simulink model "Qudcopter"  (R2021a)
settings: Solver=VariableStepAuto  StartTime=0.0  StopTime=40  RelTol=1e-3
values from neighbouring files (symbols this model uses):
  CS =     [CS.mat]    (also in Quad_dynamics.m = block.DialogPrm(1).Data)
libraries: simulink_extras x3, simulink x1
settings Model: Creator=gulso  LastModifiedBy=gulso
settings DataIOCC: SaveFormat=Structure  SignalLogging=off  DSMLogging=off  ReturnWorkspaceOutputs=off

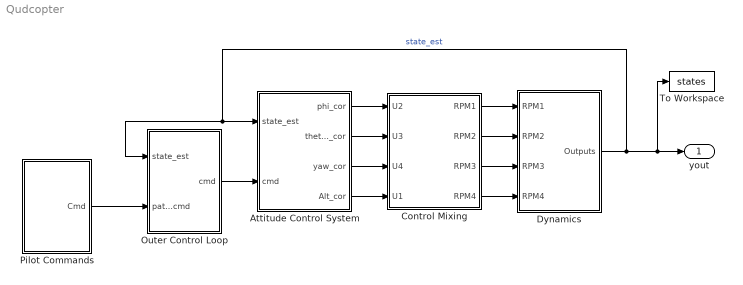
== system Qudcopter ==
  Attitude Control System : Subsystem
  "Control Mixing " : Subsystem
  Dynamics : Subsystem
  Outer Control Loop : Subsystem  mask{Kp=0.32, Ki=0.01, Kd=0.05}
      mask TypeOptions Kp: Kp1/Gain
      mask TypeOptions Ki: Ki/Gain
      mask TypeOptions Kd: Kd1/Gain
  Pilot Commands : Subsystem
  To Workspace : ToWorkspace  VariableName=states  SaveFormat=Timeseries  SampleTime=-1
      settings: Save2DSignal=2-D array (concatenate along first dimension)
  yout : Outport
  wires:
  Attitude Control System/3(yaw_cor) -> "Control Mixing "/3(U4)
  Attitude Control System/1(phi_cor) -> "Control Mixing "/1(U2)
  "Control Mixing "/3(RPM3) -> Dynamics/3(RPM3)
  Dynamics/1(Outputs) -> Attitude Control System/1(state_est), Outer Control Loop/1(state_est), yout/1, To Workspace/1  "state_est"
  "Control Mixing "/4(RPM4) -> Dynamics/4(RPM4)
  "Control Mixing "/2(RPM2) -> Dynamics/2(RPM2)
  "Control Mixing "/1(RPM1) -> Dynamics/1(RPM1)
  Outer Control Loop/1(cmd) -> Attitude Control System/2(cmd)
  Pilot Commands/1(Cmd) -> Outer Control Loop/2(path_cmd)
  Attitude Control System/2(theta_cor) -> "Control Mixing "/2(U3)
  Attitude Control System/4(Alt_cor) -> "Control Mixing "/4(U1)

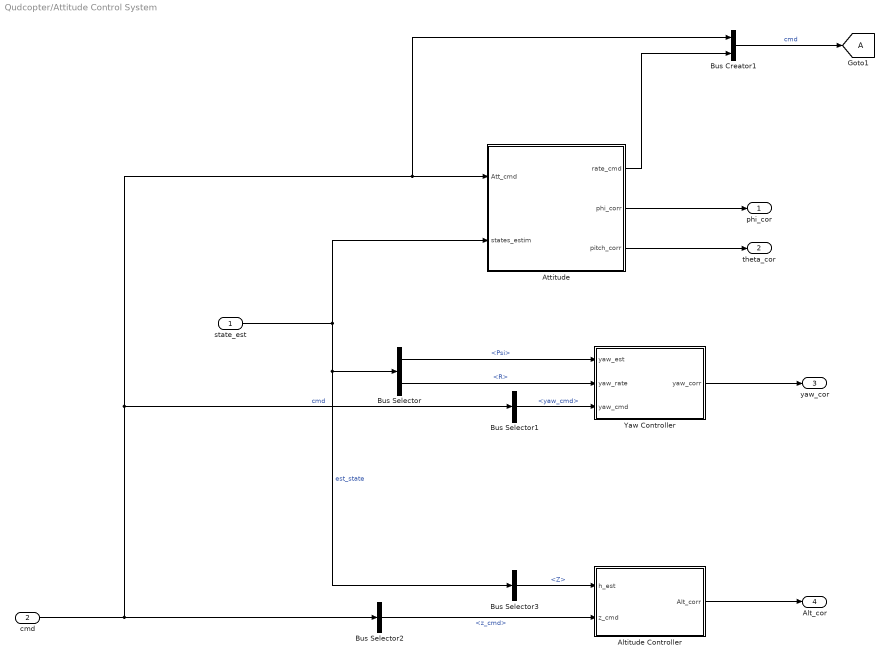
== system Qudcopter/Attitude Control System ==
  state_est : Inport
  cmd : Inport  Port=2
  Altitude Controller : Subsystem  mask{Kp=10, Ki=4, Kd=8}
      mask TypeOptions Kp: Gain/Gain
      mask TypeOptions Ki: Gain1/Gain
      mask TypeOptions Kd: Gain2/Gain
  Attitude : Subsystem  mask{Kp=2.4, Ki=1.1, Kd=1.8, Ki2=0.5}
      mask TypeOptions Kp: Kp1/Gain
      mask TypeOptions Ki: Ki1/Gain
      mask TypeOptions Kd: Kd1/Gain
      mask TypeOptions Ki2: Gainki/Gain
  Bus Creator1 : BusCreator  Inputs=2
  Bus Selector : BusSelector  OutputSignals=Psi,R
  Bus Selector1 : BusSelector  OutputSignals=pos_cmd.yaw_cmd
  Bus Selector2 : BusSelector  OutputSignals=pos_cmd.z_cmd
  Bus Selector3 : BusSelector  OutputSignals=Z
  Yaw Controller : Subsystem  mask{Kp=12, Ki=4, Kd=6}
      mask TypeOptions Kp: Gain/Gain
      mask TypeOptions Ki: Gain1/Gain
      mask TypeOptions Kd: Gain2/Gain
  phi_cor : Outport
  theta_cor : Outport  Port=2
  yaw_cor : Outport  Port=3
  Alt_cor : Outport  Port=4
  tag scope: A=global
  wires:
  Altitude Controller/1(Alt_corr) -> Alt_cor/1
  state_est/1 -> Attitude/2(states_estim), Bus Selector3/1, Bus Selector/1  "est_state"
  Bus Selector/1 -> Yaw Controller/1(yaw_est)  "<Psi>"
  Bus Selector/2 -> Yaw Controller/2(yaw_rate)  "<R>"
  cmd/1 -> Bus Selector2/1, Bus Creator1/1, Attitude/1(Att_cmd), Bus Selector1/1  "cmd"
  Bus Selector1/1 -> Yaw Controller/3(yaw_cmd)  "<yaw_cmd>"
  Bus Selector2/1 -> Altitude Controller/2(z_cmd)  "<z_cmd>"
  Bus Selector3/1 -> Altitude Controller/1(h_est)  "<Z>"
  Attitude/1(rate_cmd) -> Bus Creator1/2
  Attitude/2(phi_corr) -> phi_cor/1
  Attitude/3(pitch_corr) -> theta_cor/1
  Yaw Controller/1(yaw_corr) -> yaw_cor/1
  Bus Creator1/1 -> [A]  "cmd"

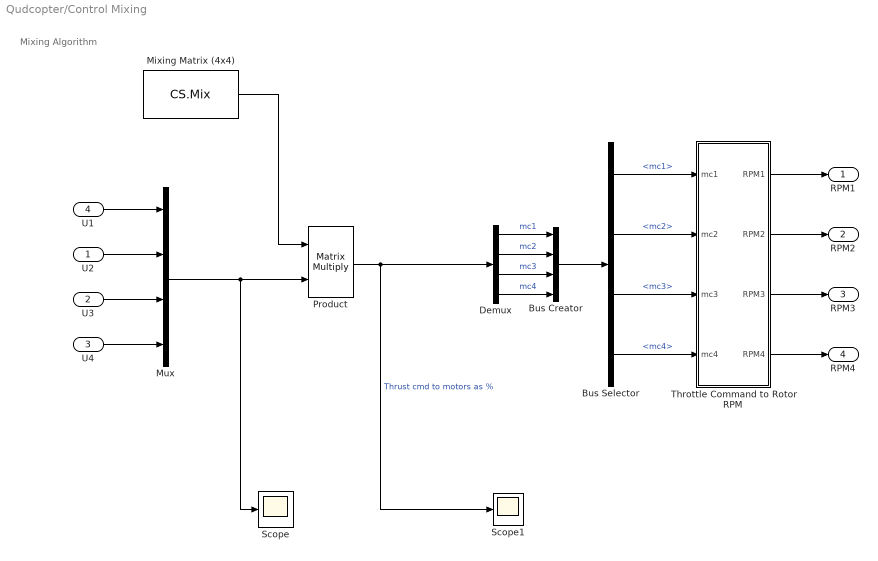
== system Qudcopter/Control Mixing  ==
  note: Mixing Algorithm
  U2 : Inport
  U3 : Inport  Port=2
  U4 : Inport  Port=3
  U1 : Inport  Port=4
  Bus Creator : BusCreator  Inputs=4
  Bus Selector : BusSelector  OutputSignals=mc1,mc2,mc3,mc4
  Demux : Demux
  Mixing Matrix (4x4) : Constant  Value=CS.Mix  OutDataTypeStr=single
  Mux : Mux
  Product : Product  Multiplication=Matrix(*)  RndMeth=Zero
  Scope : Scope
  Scope1 : Scope
  Throttle Command to Rotor RPM : Subsystem
  RPM1 : Outport
  RPM2 : Outport  Port=2
  RPM3 : Outport  Port=3
  RPM4 : Outport  Port=4
  wires:
  Throttle Command to Rotor RPM/4(RPM4) -> RPM4/1
  Throttle Command to Rotor RPM/3(RPM3) -> RPM3/1
  Throttle Command to Rotor RPM/1(RPM1) -> RPM1/1
  Throttle Command to Rotor RPM/2(RPM2) -> RPM2/1
  Bus Selector/4 -> Throttle Command to Rotor RPM/4(mc4)  "<mc4>"
  Product/1 -> Demux/1, Scope1/1  "Thrust cmd to motors as %"
  Demux/3 -> Bus Creator/3  "mc3"
  U2/1 -> Mux/2
  Mixing Matrix (4x4)/1 -> Product/1
  Bus Selector/1 -> Throttle Command to Rotor RPM/1(mc1)  "<mc1>"
  U3/1 -> Mux/3
  Demux/1 -> Bus Creator/1  "mc1"
  Demux/4 -> Bus Creator/4  "mc4"
  Bus Selector/3 -> Throttle Command to Rotor RPM/3(mc3)  "<mc3>"
  U4/1 -> Mux/4
  Demux/2 -> Bus Creator/2  "mc2"
  Bus Selector/2 -> Throttle Command to Rotor RPM/2(mc2)  "<mc2>"
  Bus Creator/1 -> Bus Selector/1
  U1/1 -> Mux/1
  Mux/1 -> Scope/1, Product/2

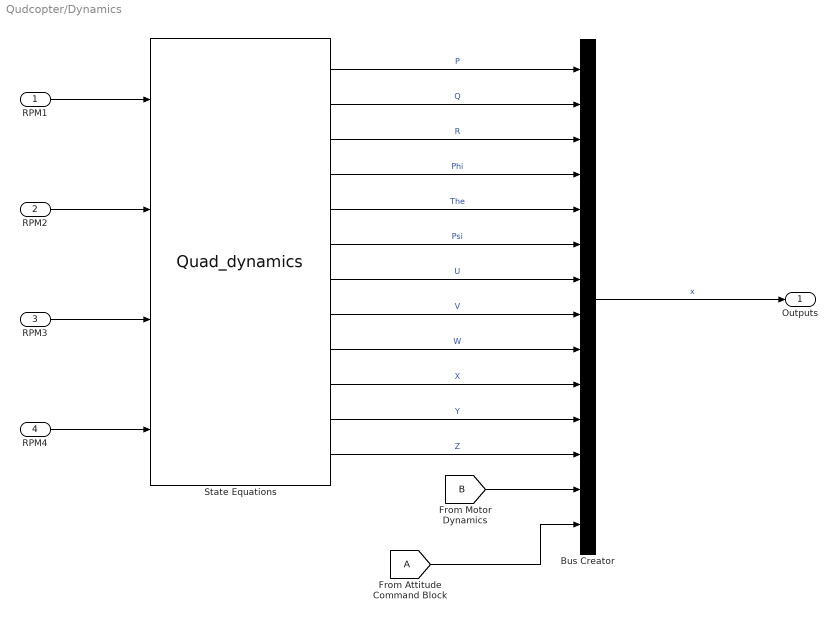
== system Qudcopter/Dynamics ==
  RPM1 : Inport
  RPM2 : Inport  Port=2
  RPM3 : Inport  Port=3
  RPM4 : Inport  Port=4
  Bus Creator : BusCreator  Inputs=14
  State Equations : M-S-Function  FunctionName=Quad_dynamics  Parameters=CS
      mask Display:
      | port_label('input', 1, 'RPM1')
      | port_label('input', 2, 'RPM2')
      | port_label('input', 3, 'RPM3')
      | port_label('input', 4, 'RPM4')
      | port_label('output', 1, 'P')
      | port_label('output', 2, 'Q')
      | port_label('output', 3, 'R')
      | port_label('output', 4, 'Phi')
      | port_label('output', 5, 'The')
      | port_label('output', 6, 'Psi')
      | port_label('output', 7, 'U')
      | port_label('output', 8, 'V')
      | port_label('output', 9, 'W')
      | port_label('output', 10, 'X')
      | port_label('output', 11, 'Y')
      | port_label('output', 12, 'Z')
  Outputs : Outport
  wires:
  State Equations/3 -> Bus Creator/3  "R"
  State Equations/1 -> Bus Creator/1  "P"
  State Equations/10 -> Bus Creator/10  "X"
  State Equations/5 -> Bus Creator/5  "The"
  State Equations/2 -> Bus Creator/2  "Q"
  State Equations/6 -> Bus Creator/6  "Psi"
  State Equations/7 -> Bus Creator/7  "U"
  State Equations/4 -> Bus Creator/4  "Phi"
  State Equations/11 -> Bus Creator/11  "Y"
  State Equations/9 -> Bus Creator/9  "W"
  State Equations/8 -> Bus Creator/8  "V"
  [B] -> Bus Creator/13
  Bus Creator/1 -> Outputs/1  "x"
  [A] -> Bus Creator/14
  State Equations/12 -> Bus Creator/12  "Z"
  RPM1/1 -> State Equations/1
  RPM2/1 -> State Equations/2
  RPM3/1 -> State Equations/3
  RPM4/1 -> State Equations/4

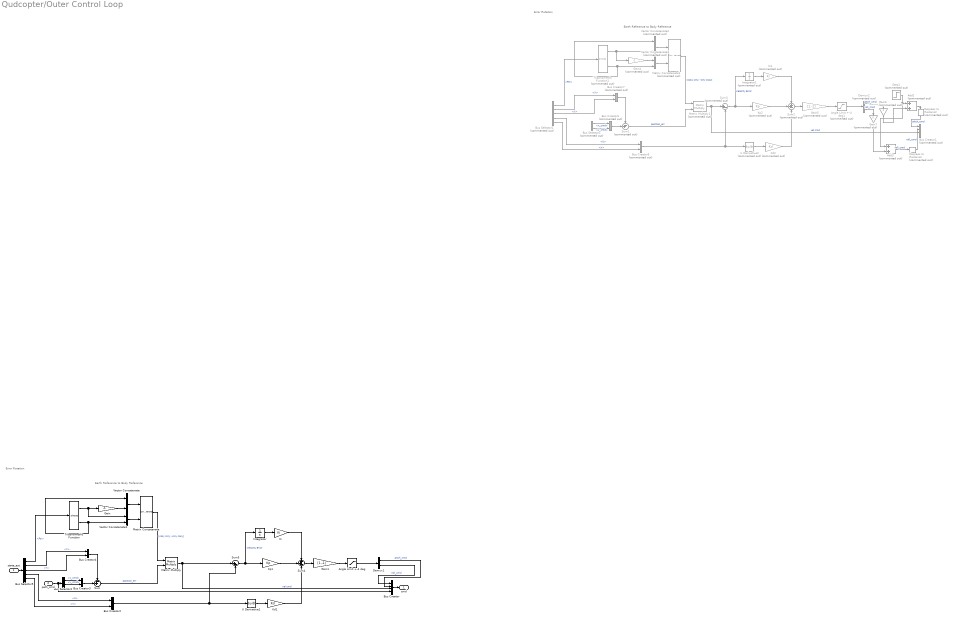
== system Qudcopter/Outer Control Loop ==
  note: Earth Reference to Body Reference
  note: Error Rotation
  note: Error Rotation
  note: Earth Reference to Body Reference
  state_est : Inport
  path_cmd : Inport  Port=2
  Add2 : Sum  Commented=on
  Add3 : Sum  Commented=on
  Angle Limit +-4 deg : Saturate  UpperLimit=4*pi/180  LowerLimit=-4*pi/180
  Angle Limit +-4 deg1 : Saturate  Commented=on  UpperLimit=4*pi/180  LowerLimit=-4*pi/180
  Bus Creator : BusCreator  Inputs=4
  Bus Creator1 : BusCreator  Commented=on  Inputs=4
  Bus Creator2 : BusCreator  Inputs=2
  Bus Creator3 : BusCreator  Inputs=2
  Bus Creator4 : BusCreator  Inputs=2
  Bus Creator5 : BusCreator  Commented=on  Inputs=2
  Bus Creator6 : BusCreator  Commented=on  Inputs=2
  Bus Creator7 : BusCreator  Commented=on  Inputs=2
  Bus Selector1 : BusSelector  Commented=on  OutputSignals=x_cmd,y_cmd
  Bus Selector2 : BusSelector  Commented=on  OutputSignals=Psi,X,Y,U,V
  Bus Selector4 : BusSelector  OutputSignals=x_cmd,y_cmd
  Bus Selector5 : BusSelector  OutputSignals=Psi,X,Y,U,V
  Degrees to Radians2 : simulink_extras/Transformations/Degrees to Radians  Commented=on
  Degrees to Radians3 : simulink_extras/Transformations/Degrees to Radians  Commented=on
  Demux1 : Demux  Outputs=2
  Demux2 : Demux  Commented=on  Outputs=2
  Gain : Gain  Gain=-1
  Gain1 : Gain  Gain=[1,-1]
  Gain4 : Gain  Commented=on  Gain=-1
  Gain5 : Gain  Commented=on  Gain=[1,-1]
  Gain6 : Gain  Commented=on  Gain=0
  Gain7 : Gain  Commented=on  Gain=0
  Integrator : Integrator  LimitOutput=on  UpperSaturationLimit=1  LowerSaturationLimit=-1
  Integrator1 : Integrator  Commented=on  LimitOutput=on  UpperSaturationLimit=1  LowerSaturationLimit=-1
  Kd1 : Gain  Gain=Kd
  Kd2 : Gain  Commented=on  Gain=Kd
  Ki : Gain  Gain=Ki
  Ki1 : Gain  Commented=on  Gain=Ki
  Kp1 : Gain  Gain=Kp
  Kp2 : Gain  Commented=on  Gain=Kp
  Matrix Concatenate : Concatenate  Mode=Multidimensional array  ConcatenateDimension=2
  Matrix Concatenate1 : Concatenate  Commented=on  Mode=Multidimensional array  ConcatenateDimension=2
  Matrix Multiply : Product  Multiplication=Matrix(*)
  Matrix Multiply1 : Product  Commented=on  Multiplication=Matrix(*)
  Step1 : Step  Commented=on  SampleTime=0
  Sum : Sum  Inputs=-+|
  Sum1 : Sum  Commented=on  Inputs=-+|
  Sum2 : Sum  Commented=on  Inputs=++-
  Sum3 : Sum  Commented=on  Inputs=|+-
  Sum4 : Sum  Inputs=++-
  Sum5 : Sum  Inputs=|+-
  Trigonometric Function : Trigonometry  Operator=sincos
  Trigonometric Function1 : Trigonometry  Commented=on  Operator=sincos
  U Derivative1 : Derivative
  U Derivative2 : Derivative  Commented=on
  Vector Concatenate : Concatenate
  Vector Concatenate1 : Concatenate
  Vector Concatenate2 : Concatenate  Commented=on
  Vector Concatenate3 : Concatenate  Commented=on
  cmd : Outport
  wires:
  Bus Selector5/1 -> Trigonometric Function/1  "<Psi>"
  state_est/1 -> Bus Selector5/1
  Bus Selector5/2 -> Bus Creator4/1  "<X>"
  Bus Selector5/5 -> Bus Creator2/2  "<V>"
  Bus Selector4/1 -> Bus Creator3/1  "<x_cmd>"
  Demux1/2 -> Bus Creator/1  "roll_cmd"
  Bus Selector4/2 -> Bus Creator3/2  "<y_cmd>"
  Bus Selector5/4 -> Bus Creator2/1  "<U>"
  Bus Selector5/3 -> Bus Creator4/2  "<Y>"
  path_cmd/1 -> Bus Creator/4, Bus Selector4/1
  Matrix Multiply/1 -> Bus Creator/3, Sum5/1  "vel cmd"
  Bus Creator/1 -> cmd/1
  Kp1/1 -> Sum4/2
  Sum5/1 -> Integrator/1, Kp1/1  "Velocity Error"
  Sum/1 -> Matrix Multiply/2  "position_err"
  Ki/1 -> Sum4/1
  Integrator/1 -> Ki/1
  Angle Limit +-4 deg/1 -> Demux1/1
  Gain1/1 -> Angle Limit +-4 deg/1
  Sum4/1 -> Gain1/1
  Kd1/1 -> Sum4/3
  Bus Creator2/1 -> U Derivative1/1, Sum5/2
  U Derivative1/1 -> Kd1/1
  Bus Creator4/1 -> Sum/1
  Bus Creator3/1 -> Sum/2
  Vector Concatenate/1 -> Matrix Concatenate/1
  Vector Concatenate1/1 -> Matrix Concatenate/2
  Trigonometric Function/1 -> Vector Concatenate1/1, Gain/1
  Matrix Concatenate/1 -> Matrix Multiply/1  "[cosy siny; -siny cosy]"
  Trigonometric Function/2 -> Vector Concatenate1/2, Vector Concatenate/1
  Gain6/1 -> Add2/2
  Add2/1 -> Degrees to Radians2/1
  Demux2/1 -> Gain6/1  "pitch_cmd"
  Add3/1 -> Degrees to Radians3/1  "roll_cmd"
  Demux2/2 -> Gain7/1  "roll_cmd"
  Trigonometric Function1/1 -> Vector Concatenate2/2, Gain4/1
  Trigonometric Function1/2 -> Vector Concatenate3/2, Vector Concatenate2/1
  Vector Concatenate2/1 -> Matrix Concatenate1/1
  Bus Creator6/1 -> Sum1/2
  Step1/1 -> Add3/1, Add2/1
  Bus Creator7/1 -> Sum1/1
  ? -> Bus Creator1/4, Bus Selector1/1
  Integrator1/1 -> Ki1/1
  Matrix Concatenate1/1 -> Matrix Multiply1/1  "[cosy siny; -siny cosy]"
  Kd2/1 -> Sum2/3
  Bus Creator5/1 -> U Derivative2/1, Sum3/2
  Bus Selector2/4 -> Bus Creator5/1  "<U>"
  Angle Limit +-4 deg1/1 -> Demux2/1
  Sum2/1 -> Gain5/1
  Degrees to Radians2/1 -> Bus Creator1/1  "pitch_cmd"
  Gain5/1 -> Angle Limit +-4 deg1/1
  Vector Concatenate3/1 -> Matrix Concatenate1/2
  Bus Selector2/3 -> Bus Creator7/2  "<Y>"
  Ki1/1 -> Sum2/1
  Sum1/1 -> Matrix Multiply1/2  "position_err"
  Sum3/1 -> Integrator1/1, Kp2/1  "Velocity Error"
  Gain7/1 -> Add3/2
  Matrix Multiply1/1 -> Bus Creator1/3, Sum3/1  "vel cmd"
  U Derivative2/1 -> Kd2/1
  Bus Selector2/1 -> Trigonometric Function1/1  "<Psi>"
  Kp2/1 -> Sum2/2
  Gain4/1 -> Vector Concatenate3/1
  Bus Selector2/5 -> Bus Creator5/2  "<V>"
  Bus Selector1/2 -> Bus Creator6/2  "<y_cmd>"
  Degrees to Radians3/1 -> Bus Creator1/2  "roll_cmd"
  ? -> Bus Selector2/1
  Bus Selector1/1 -> Bus Creator6/1  "<x_cmd>"
  Bus Selector2/2 -> Bus Creator7/1  "<X>"
  Demux1/1 -> Bus Creator/2  "pitch_cmd"
  Gain/1 -> Vector Concatenate/2

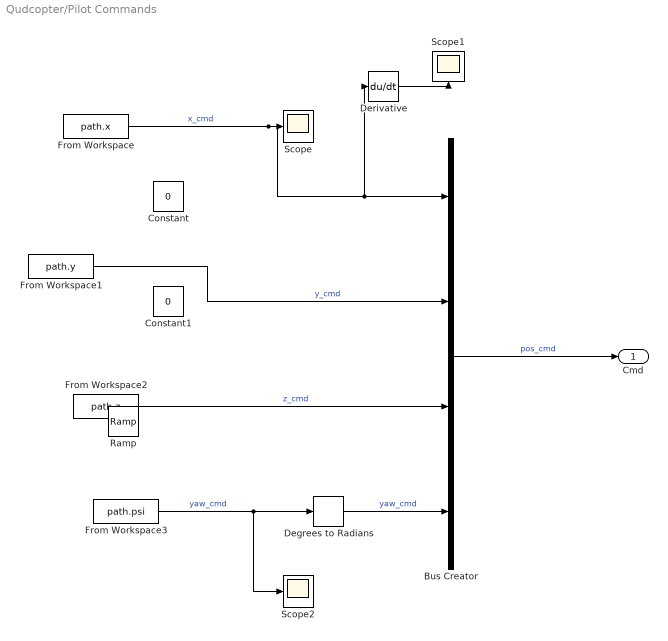
== system Qudcopter/Pilot Commands ==
  Bus Creator : BusCreator  Inputs=4
  Constant : Constant  Value=0
  Constant1 : Constant  Value=0
  Degrees to Radians : simulink_extras/Transformations/Degrees to Radians
  Derivative : Derivative
  From Workspace : FromWorkspace  VariableName=path.x
  From Workspace1 : FromWorkspace  VariableName=path.y
  From Workspace2 : FromWorkspace  VariableName=path.z
  From Workspace3 : FromWorkspace  VariableName=path.psi
  Ramp : simulink/Sources/Ramp  slope=1  start=0  InitialOutput=0
  Scope : Scope
  Scope1 : Scope
  Scope2 : Scope
  Cmd : Outport
  wires:
  Bus Creator/1 -> Cmd/1  "pos_cmd"
  Degrees to Radians/1 -> Bus Creator/4  "yaw_cmd"
  From Workspace/1 -> Derivative/1, Bus Creator/1, Scope/1  "x_cmd"
  From Workspace1/1 -> Bus Creator/2  "y_cmd"
  Derivative/1 -> Scope1/1
  From Workspace3/1 -> Scope2/1, Degrees to Radians/1  "yaw_cmd"
  From Workspace2/1 -> Bus Creator/3  "z_cmd"

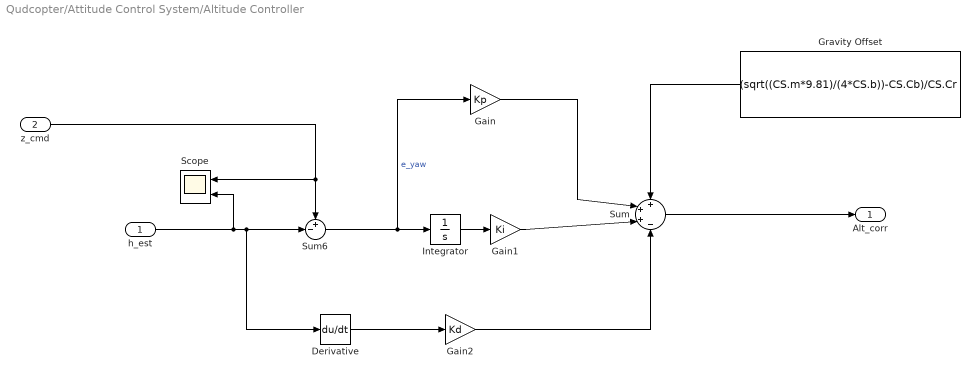
== system Qudcopter/Attitude Control System/Altitude Controller ==
  h_est : Inport
  z_cmd : Inport  Port=2
  Derivative : Derivative
  Gain : Gain  Gain=Kp
  Gain1 : Gain  Gain=Ki
  Gain2 : Gain  Gain=Kd
  Gravity Offset : Constant  Value=(sqrt((CS.m*9.81)/(4*CS.b))-CS.Cb)/CS.Cr  VectorParams1D=off
  Integrator : Integrator  LimitOutput=on  UpperSaturationLimit=1  LowerSaturationLimit=-1
  Scope : Scope  NumInputPorts=2
  Sum : Sum  Inputs=+++-
  Sum6 : Sum  Inputs=+-|
  Alt_corr : Outport
  wires:
  z_cmd/1 -> Sum6/1, Scope/1
  h_est/1 -> Scope/2, Derivative/1, Sum6/2
  Sum6/1 -> Gain/1, Integrator/1  "e_yaw"
  Gravity Offset/1 -> Sum/1
  Sum/1 -> Alt_corr/1
  Gain/1 -> Sum/2
  Integrator/1 -> Gain1/1
  Gain1/1 -> Sum/3
  Derivative/1 -> Gain2/1
  Gain2/1 -> Sum/4

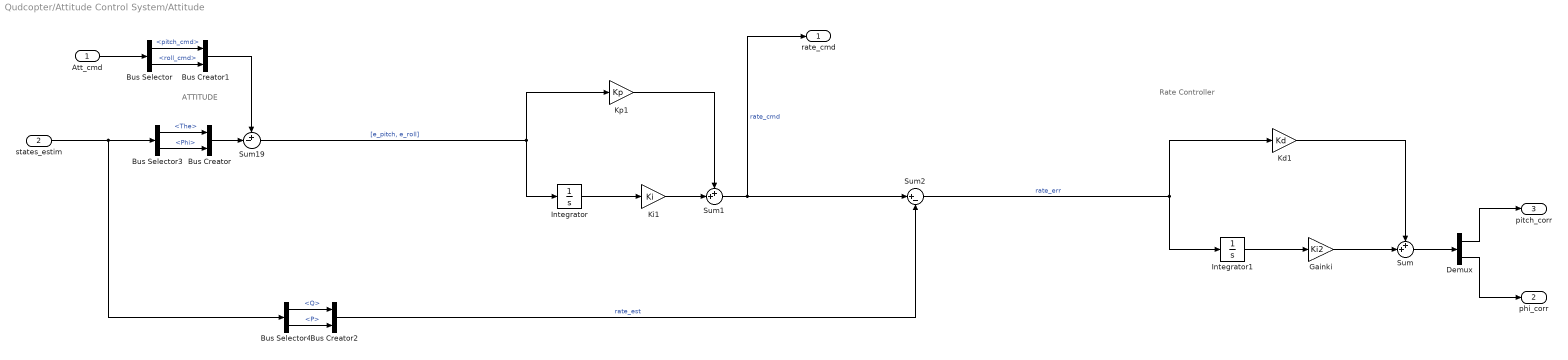
== system Qudcopter/Attitude Control System/Attitude ==
  note: Rate Controller
  note: ATTITUDE
  Att_cmd : Inport
  states_estim : Inport  Port=2
  Bus Creator : BusCreator  Inputs=2
  Bus Creator1 : BusCreator  Inputs=2
  Bus Creator2 : BusCreator  Inputs=2
  Bus Selector : BusSelector  OutputSignals=pitch_cmd,roll_cmd
  Bus Selector3 : BusSelector  OutputSignals=The,Phi
  Bus Selector4 : BusSelector  OutputSignals=Q,P
  Demux : Demux  Outputs=2
  Gainki : Gain  Gain=Ki2
  Integrator : Integrator  LimitOutput=on  UpperSaturationLimit=1  LowerSaturationLimit=-1
  Integrator1 : Integrator  LimitOutput=on  UpperSaturationLimit=1  LowerSaturationLimit=-1
  Kd1 : Gain  Gain=Kd
  Ki1 : Gain  Gain=Ki
  Kp1 : Gain  Gain=Kp
  Sum : Sum  Inputs=++|
  Sum1 : Sum  Inputs=++|
  Sum19 : Sum  Inputs=+-|
  Sum2 : Sum  Inputs=|+-
  rate_cmd : Outport
  phi_corr : Outport  Port=2  VectorParamsAs1DForOutWhenUnconnected=off
  pitch_corr : Outport  Port=3  VectorParamsAs1DForOutWhenUnconnected=off
  wires:
  Bus Selector3/2 -> Bus Creator/2  "<Phi>"
  states_estim/1 -> Bus Selector4/1, Bus Selector3/1
  Bus Creator/1 -> Sum19/2
  Bus Selector3/1 -> Bus Creator/1  "<The>"
  Sum19/1 -> Kp1/1, Integrator/1  "[e_pitch, e_roll]"
  Integrator/1 -> Ki1/1
  Kp1/1 -> Sum1/1
  Ki1/1 -> Sum1/2
  Att_cmd/1 -> Bus Selector/1
  Bus Selector/2 -> Bus Creator1/2  "<roll_cmd>"
  Bus Selector/1 -> Bus Creator1/1  "<pitch_cmd>"
  Bus Creator1/1 -> Sum19/1
  Bus Selector4/1 -> Bus Creator2/1  "<Q>"
  Bus Selector4/2 -> Bus Creator2/2  "<P>"
  Sum2/1 -> Integrator1/1, Kd1/1  "rate_err"
  Demux/1 -> pitch_corr/1
  Demux/2 -> phi_corr/1
  Sum/1 -> Demux/1
  Kd1/1 -> Sum/1
  Gainki/1 -> Sum/2
  Integrator1/1 -> Gainki/1
  Bus Creator2/1 -> Sum2/2  "rate_est"
  Sum1/1 -> Sum2/1, rate_cmd/1  "rate_cmd"

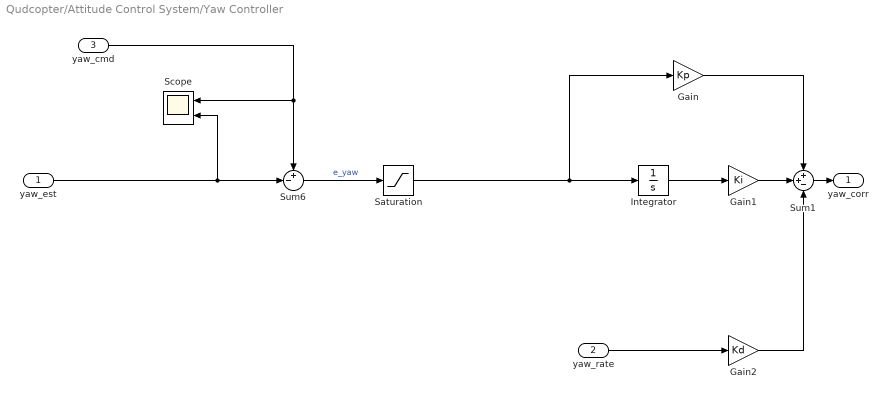
== system Qudcopter/Attitude Control System/Yaw Controller ==
  yaw_est : Inport
  yaw_rate : Inport  Port=2
  yaw_cmd : Inport  Port=3
  Gain : Gain  Gain=Kp
  Gain1 : Gain  Gain=Ki
  Gain2 : Gain  Gain=Kd
  Integrator : Integrator  LimitOutput=on  UpperSaturationLimit=1  LowerSaturationLimit=-1
  Saturation : Saturate  UpperLimit=pi  LowerLimit=-pi
  Scope : Scope  NumInputPorts=2
  Sum1 : Sum  Inputs=++-
  Sum6 : Sum  Inputs=+-|
  yaw_corr : Outport
  wires:
  yaw_cmd/1 -> Sum6/1, Scope/1
  Gain/1 -> Sum1/1
  Integrator/1 -> Gain1/1
  Gain2/1 -> Sum1/3
  yaw_rate/1 -> Gain2/1
  Sum6/1 -> Saturation/1  "e_yaw"
  Gain1/1 -> Sum1/2
  yaw_est/1 -> Sum6/2, Scope/2
  Sum1/1 -> yaw_corr/1
  Saturation/1 -> Integrator/1, Gain/1

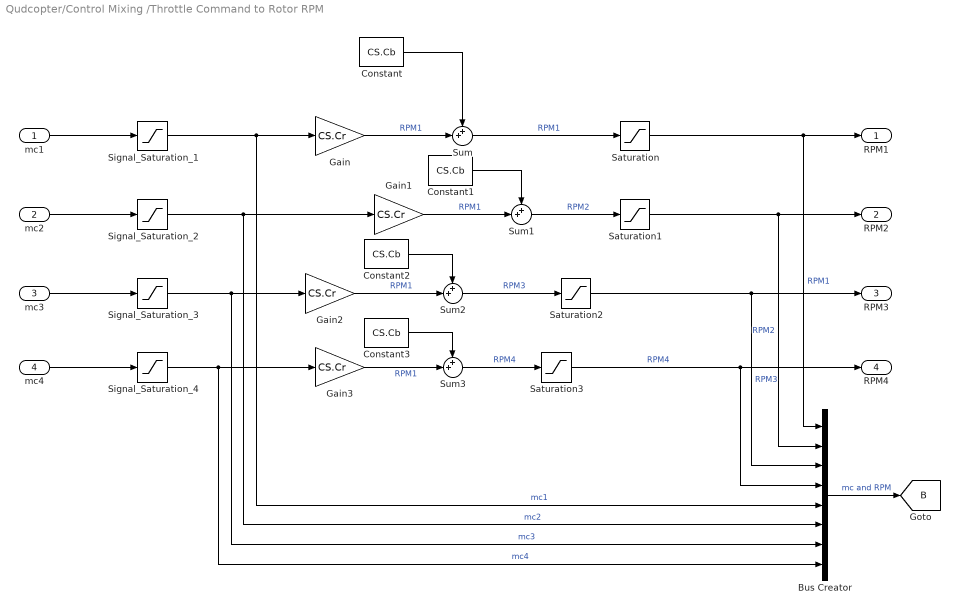
== system Qudcopter/Control Mixing /Throttle Command to Rotor RPM ==
  mc1 : Inport
  mc2 : Inport  Port=2
  mc3 : Inport  Port=3
  mc4 : Inport  Port=4
  Bus Creator : BusCreator  Inputs=8
  Constant{,1..3} (4 alike) : Constant  Value=CS.Cb
  Gain{,1..3} (4 alike) : Gain  Gain=CS.Cr
  Saturation{,1..3} (4 alike) : Saturate  UpperLimit=10e3  LowerLimit=CS.Cb
  Signal_Saturation_{1..4} (4 alike) : Saturate  UpperLimit=100  LowerLimit=0
  Sum{,1..3} (4 alike) : Sum  Inputs=++|
  RPM1 : Outport
  RPM2 : Outport  Port=2
  RPM3 : Outport  Port=3
  RPM4 : Outport  Port=4
  tag scope: B=global
  wires:
  Signal_Saturation_1/1 -> Bus Creator/5, Gain/1  "mc1"
  mc1/1 -> Signal_Saturation_1/1
  Signal_Saturation_4/1 -> Gain3/1, Bus Creator/8  "mc4"
  mc4/1 -> Signal_Saturation_4/1
  Signal_Saturation_3/1 -> Gain2/1, Bus Creator/7  "mc3"
  Sum2/1 -> Saturation2/1  "RPM3"
  Signal_Saturation_2/1 -> Gain1/1, Bus Creator/6  "mc2"
  Saturation3/1 -> Bus Creator/4, RPM4/1  "RPM4"
  Sum/1 -> Saturation/1  "RPM1"
  mc2/1 -> Signal_Saturation_2/1
  Sum1/1 -> Saturation1/1  "RPM2"
  Bus Creator/1 -> [B]  "mc and RPM"
  mc3/1 -> Signal_Saturation_3/1
  Gain/1 -> Sum/2  "RPM1"
  Constant/1 -> Sum/1
  Constant1/1 -> Sum1/1
  Gain1/1 -> Sum1/2  "RPM1"
  Constant2/1 -> Sum2/1
  Gain2/1 -> Sum2/2  "RPM1"
  Constant3/1 -> Sum3/1
  Gain3/1 -> Sum3/2  "RPM1"
  Saturation/1 -> Bus Creator/1, RPM1/1  "RPM1"
  Saturation1/1 -> Bus Creator/2, RPM2/1  "RPM2"
  Saturation2/1 -> Bus Creator/3, RPM3/1  "RPM3"
  Sum3/1 -> Saturation3/1  "RPM4"
